simulink model "ProjectArchitecture"  (R2026a)
settings: Solver=VariableStepAuto  StopTime=100
undefined symbols (not defined in the file): Boomgate_Up, Close_Cmd, Dwn, Open, Pedestrian_Lights_On, Traffic_Lights_On
(part 1 of 2)
settings Model: DataDictionary=Architecture_DD.sldd  Creator=jaime  LastModifiedBy=jaime

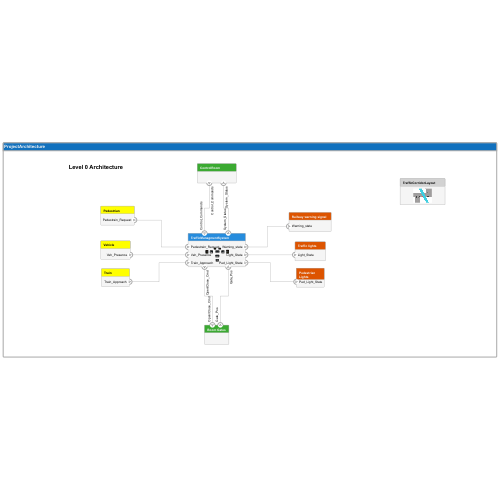
[thumbnail: Simulink's stored preview of the top-level diagram]
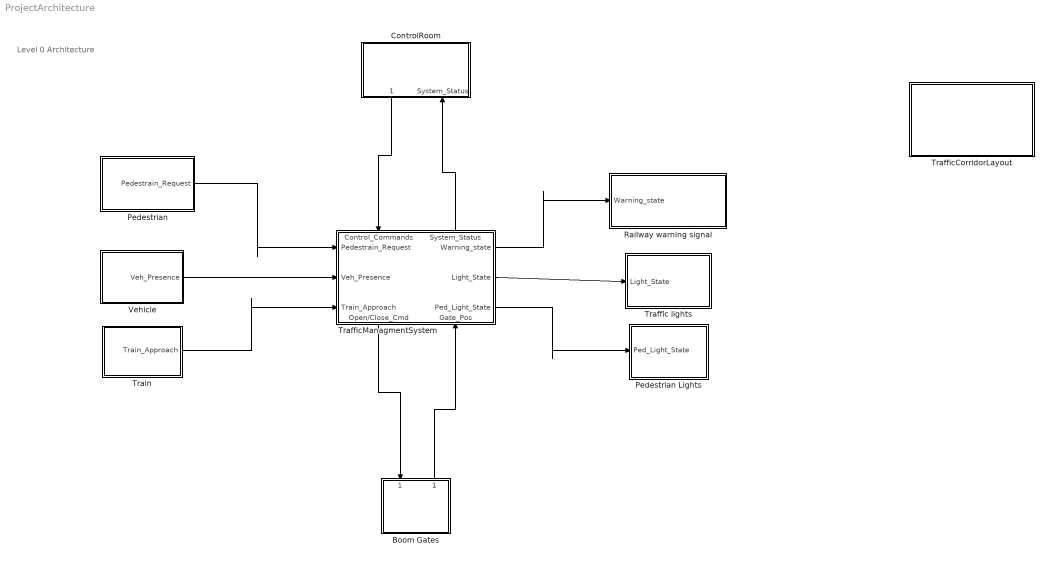
== system ProjectArchitecture ==
  note: Level 0 Architecture
  Boom Gates : Subsystem
      settings: PortSchema="{\"entries\":[{\"content\":{\"headerSize\":26,\"margin\":15,\"minimumSpacing\":25,\"sides\":[{\"content\":{},\"type\":\"ConnectorPlacement.EquallySpacedRectSide\",\"uuid\":\"97ee8f68-7c90-442c-8c58-6fb9a02436b1\"},{\"content\":{\"side\":\"RIGHT\"},\"type\":\"ConnectorPlacement.EquallySpacedRectSide\",\"uuid\":\"273d2447-c6df-49b3-a65a-924db0dbcca5\"},{\"content\":{\"connectorIds\":[\"In1\",\"Out1\"],\"side\":\"TOP\"},\"type\":\"ConnectorPlacement.EquallySpacedRectSide\",\"uuid\":\"83dd206d-8fe2-4459-a401-ead6bb37f785\"}]},\"type\":\"ConnectorPlacement.EquallySpacedConnector\",\"uuid\":\"02b69e8e-5274-42ce-be18-831f28eb2f2d\"}],\"packageUris\":[\"http://schema.mathworks.com/mf0/Connector/R2020b\"],\"version\":\"1.0\"}"
  ControlRoom : Subsystem
      settings: PortSchema="{\"entries\":[{\"content\":{\"headerSize\":26,\"margin\":15,\"minimumSpacing\":25,\"sides\":[{\"content\":{},\"type\":\"ConnectorPlacement.EquallySpacedRectSide\",\"uuid\":\"97ee8f68-7c90-442c-8c58-6fb9a02436b1\"},{\"content\":{\"side\":\"RIGHT\"},\"type\":\"ConnectorPlacement.EquallySpacedRectSide\",\"uuid\":\"273d2447-c6df-49b3-a65a-924db0dbcca5\"},{\"content\":{\"side\":\"TOP\"},\"type\":\"ConnectorPlacement.EquallySpacedRectSide\",\"uuid\":\"83dd206d-8fe2-4459-a401-ead6bb37f785\"},{\"content\":{\"connectorIds\":[\"Out1\",\"In1\"],\"side\":\"BOTTOM\"},\"type\":\"ConnectorPlacement.EquallySpacedRectSide\",\"uuid\":\"7511c607-cb92-42c1-9f90-436e19c4c1f5\"}]},\"type\":\"ConnectorPlacement.EquallySpacedConnector\",\"uuid\":\"02b69e8e-5274-42ce-be18-831f28eb2f2d\"}],\"packageUris\":[\"http://schema.mathworks.com/mf0/Connector/R2020b\"],\"version\":\"1.0\"}"
  Pedestrian : Subsystem
      settings: PortSchema="{\"entries\":[{\"content\":{\"headerSize\":26,\"margin\":15,\"minimumSpacing\":25,\"sides\":[{\"content\":{},\"type\":\"ConnectorPlacement.EquallySpacedRectSide\",\"uuid\":\"97ee8f68-7c90-442c-8c58-6fb9a02436b1\"},{\"content\":{\"connectorIds\":[\"Out1\"],\"side\":\"RIGHT\"},\"type\":\"ConnectorPlacement.EquallySpacedRectSide\",\"uuid\":\"273d2447-c6df-49b3-a65a-924db0dbcca5\"},{\"content\":{\"side\":\"TOP\"},\"type\":\"ConnectorPlacement.EquallySpacedRectSide\",\"uuid\":\"83dd206d-8fe2-4459-a401-ead6bb37f785\"}]},\"type\":\"ConnectorPlacement.EquallySpacedConnector\",\"uuid\":\"02b69e8e-5274-42ce-be18-831f28eb2f2d\"}],\"packageUris\":[\"http://schema.mathworks.com/mf0/Connector/R2020b\"],\"version\":\"1.0\"}"
  Pedestrian Lights : Subsystem
      settings: PortSchema="{\"entries\":[{\"content\":{\"headerSize\":26,\"margin\":15,\"minimumSpacing\":25,\"sides\":[{\"content\":{\"connectorIds\":[\"In1\"]},\"type\":\"ConnectorPlacement.EquallySpacedRectSide\",\"uuid\":\"97ee8f68-7c90-442c-8c58-6fb9a02436b1\"},{\"content\":{\"side\":\"RIGHT\"},\"type\":\"ConnectorPlacement.EquallySpacedRectSide\",\"uuid\":\"273d2447-c6df-49b3-a65a-924db0dbcca5\"},{\"content\":{\"side\":\"TOP\"},\"type\":\"ConnectorPlacement.EquallySpacedRectSide\",\"uuid\":\"83dd206d-8fe2-4459-a401-ead6bb37f785\"}]},\"type\":\"ConnectorPlacement.EquallySpacedConnector\",\"uuid\":\"02b69e8e-5274-42ce-be18-831f28eb2f2d\"}],\"packageUris\":[\"http://schema.mathworks.com/mf0/Connector/R2020b\"],\"version\":\"1.0\"}"
  Railway warning signal : Subsystem
      settings: PortSchema="{\"entries\":[{\"content\":{\"headerSize\":26,\"margin\":15,\"minimumSpacing\":25,\"sides\":[{\"content\":{\"connectorIds\":[\"In1\"]},\"type\":\"ConnectorPlacement.EquallySpacedRectSide\",\"uuid\":\"97ee8f68-7c90-442c-8c58-6fb9a02436b1\"},{\"content\":{\"side\":\"RIGHT\"},\"type\":\"ConnectorPlacement.EquallySpacedRectSide\",\"uuid\":\"273d2447-c6df-49b3-a65a-924db0dbcca5\"},{\"content\":{\"side\":\"TOP\"},\"type\":\"ConnectorPlacement.EquallySpacedRectSide\",\"uuid\":\"83dd206d-8fe2-4459-a401-ead6bb37f785\"}]},\"type\":\"ConnectorPlacement.EquallySpacedConnector\",\"uuid\":\"02b69e8e-5274-42ce-be18-831f28eb2f2d\"}],\"packageUris\":[\"http://schema.mathworks.com/mf0/Connector/R2020b\"],\"version\":\"1.0\"}"
  Traffic lights : Subsystem
      settings: PortSchema="{\"entries\":[{\"content\":{\"headerSize\":26,\"margin\":15,\"minimumSpacing\":25,\"sides\":[{\"content\":{\"connectorIds\":[\"In1\"]},\"type\":\"ConnectorPlacement.EquallySpacedRectSide\",\"uuid\":\"97ee8f68-7c90-442c-8c58-6fb9a02436b1\"},{\"content\":{\"side\":\"RIGHT\"},\"type\":\"ConnectorPlacement.EquallySpacedRectSide\",\"uuid\":\"273d2447-c6df-49b3-a65a-924db0dbcca5\"},{\"content\":{\"side\":\"TOP\"},\"type\":\"ConnectorPlacement.EquallySpacedRectSide\",\"uuid\":\"83dd206d-8fe2-4459-a401-ead6bb37f785\"}]},\"type\":\"ConnectorPlacement.EquallySpacedConnector\",\"uuid\":\"02b69e8e-5274-42ce-be18-831f28eb2f2d\"}],\"packageUris\":[\"http://schema.mathworks.com/mf0/Connector/R2020b\"],\"version\":\"1.0\"}"
  TrafficCorridorLayout : Subsystem
      settings: PortSchema="{\"entries\":[{\"content\":{\"headerSize\":26,\"margin\":15,\"minimumSpacing\":25,\"sides\":[{\"content\":{},\"type\":\"ConnectorPlacement.EquallySpacedRectSide\",\"uuid\":\"5e856c94-202a-4db7-8bb0-19ecc7451e2e\"},{\"content\":{\"side\":\"RIGHT\"},\"type\":\"ConnectorPlacement.EquallySpacedRectSide\",\"uuid\":\"60535048-e66e-4ce0-b527-a8381120427d\"},{\"content\":{\"side\":\"TOP\"},\"type\":\"ConnectorPlacement.EquallySpacedRectSide\",\"uuid\":\"89f0e98b-19cd-4c6c-a057-5a9848434c28\"}]},\"type\":\"ConnectorPlacement.EquallySpacedConnector\",\"uuid\":\"91963807-6f38-48ec-a453-a1c872930595\"}],\"packageUris\":[\"http://schema.mathworks.com/mf0/Connector/R2020b\"],\"version\":\"1.0\"}"
  TrafficManagmentSystem : Subsystem
      settings: PortSchema="{\"entries\":[{\"content\":{\"headerSize\":26,\"margin\":15,\"minimumSpacing\":25,\"sides\":[{\"content\":{\"connectorIds\":[\"In3\",\"In4\",\"In5\"]},\"type\":\"ConnectorPlacement.EquallySpacedRectSide\",\"uuid\":\"97ee8f68-7c90-442c-8c58-6fb9a02436b1\"},{\"content\":{\"connectorIds\":[\"Out1\",\"Out2\",\"Out3\"],\"side\":\"RIGHT\"},\"type\":\"ConnectorPlacement.EquallySpacedRectSide\",\"uuid\":\"273d2447-c6df-49b3-a65a-924db0dbcca5\"},{\"content\":{\"connectorIds\":[\"In2\",\"Out5\"],\"side\":\"TOP\"},\"type\":\"ConnectorPlacement.EquallySpacedRectSide\",\"uuid\":\"83dd206d-8fe2-4459-a401-ead6bb37f785\"},{\"content\":{\"connectorIds\":[\"Out4\",\"In1\"],\"side\":\"BOTTOM\"},\"type\":\"ConnectorPlacement.EquallySpacedRectSide\",\"uuid\":\"d3110f55-67a6-4d73-b0ad-816204b8dc40\"}]},\"type\":\"ConnectorPlacement.EquallySpacedConnector\",\"uuid\":\"02b69e8e-5274-42ce-be18-831f28eb2f2d\"}],\"packageUris\":[\"http://schema.mathworks.com/mf0/Connector/R2020b\"],\"version\":\"1.0\"}"
  Train : Subsystem
      settings: PortSchema="{\"entries\":[{\"content\":{\"headerSize\":26,\"margin\":15,\"minimumSpacing\":25,\"sides\":[{\"content\":{},\"type\":\"ConnectorPlacement.EquallySpacedRectSide\",\"uuid\":\"97ee8f68-7c90-442c-8c58-6fb9a02436b1\"},{\"content\":{\"connectorIds\":[\"Out1\"],\"side\":\"RIGHT\"},\"type\":\"ConnectorPlacement.EquallySpacedRectSide\",\"uuid\":\"273d2447-c6df-49b3-a65a-924db0dbcca5\"},{\"content\":{\"side\":\"TOP\"},\"type\":\"ConnectorPlacement.EquallySpacedRectSide\",\"uuid\":\"83dd206d-8fe2-4459-a401-ead6bb37f785\"}]},\"type\":\"ConnectorPlacement.EquallySpacedConnector\",\"uuid\":\"02b69e8e-5274-42ce-be18-831f28eb2f2d\"}],\"packageUris\":[\"http://schema.mathworks.com/mf0/Connector/R2020b\"],\"version\":\"1.0\"}"
  Vehicle : Subsystem
      settings: PortSchema="{\"entries\":[{\"content\":{\"headerSize\":26,\"margin\":15,\"minimumSpacing\":25,\"sides\":[{\"content\":{},\"type\":\"ConnectorPlacement.EquallySpacedRectSide\",\"uuid\":\"97ee8f68-7c90-442c-8c58-6fb9a02436b1\"},{\"content\":{\"connectorIds\":[\"Out1\"],\"side\":\"RIGHT\"},\"type\":\"ConnectorPlacement.EquallySpacedRectSide\",\"uuid\":\"273d2447-c6df-49b3-a65a-924db0dbcca5\"},{\"content\":{\"side\":\"TOP\"},\"type\":\"ConnectorPlacement.EquallySpacedRectSide\",\"uuid\":\"83dd206d-8fe2-4459-a401-ead6bb37f785\"}]},\"type\":\"ConnectorPlacement.EquallySpacedConnector\",\"uuid\":\"02b69e8e-5274-42ce-be18-831f28eb2f2d\"}],\"packageUris\":[\"http://schema.mathworks.com/mf0/Connector/R2020b\"],\"version\":\"1.0\"}"
  wires:
  Pedestrian/1(Pedestrain_Request) -> TrafficManagmentSystem/3(Pedestrain_Request)
  Train/1(Train_Approach) -> TrafficManagmentSystem/5(Train_Approach)
  ControlRoom/1(Control_Commands) -> TrafficManagmentSystem/2(Control_Commands)
  TrafficManagmentSystem/5(System_Status) -> ControlRoom/1(System_Status)
  TrafficManagmentSystem/4(Open/Close_Cmd) -> Boom Gates/1(Open/Close_Cmd)
  TrafficManagmentSystem/3(Ped_Light_State) -> Pedestrian Lights/1(Ped_Light_State)
  TrafficManagmentSystem/2(Light_State) -> Traffic lights/1(Light_State)
  Boom Gates/1(Gate_Pos) -> TrafficManagmentSystem/1(Gate_Pos)
  TrafficManagmentSystem/1(Warning_state) -> Railway warning signal/1(Warning_state)
  Vehicle/1(Veh_Presence) -> TrafficManagmentSystem/4(Veh_Presence)

== system ProjectArchitecture/Boom Gates ==
  Bus Element In1 : Inport  PortName=Open/Close_Cmd
  Bus Element Out1 : Outport  PortName=Gate_Pos

== system ProjectArchitecture/ControlRoom ==
  Bus Element In1 : Inport  PortName=System_Status
  Bus Element Out1 : Outport  PortName=Control_Commands

== system ProjectArchitecture/Pedestrian ==
  Bus Element Out1 : Outport  PortName=Pedestrain_Request

== system ProjectArchitecture/Pedestrian Lights ==
  Bus Element In1 : Inport  PortName=Ped_Light_State

== system ProjectArchitecture/Railway warning signal ==
  Bus Element In1 : Inport  PortName=Warning_state

== system ProjectArchitecture/Traffic lights ==
  Bus Element In1 : Inport  PortName=Light_State

== system ProjectArchitecture/TrafficCorridorLayout ==

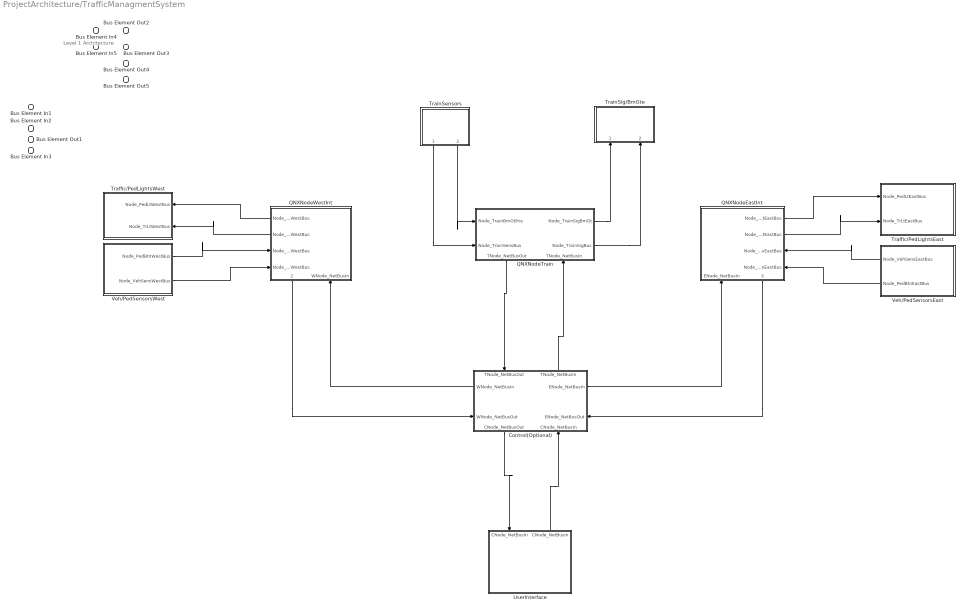
== system ProjectArchitecture/TrafficManagmentSystem ==
  note: Level 1 Architecture
  Bus Element In5 : Inport  PortName=Gate_Pos
  Bus Element In4 : Inport  Port=2  PortName=Control_Commands
  Bus Element In1 : Inport  Port=3  PortName=Pedestrain_Request
  Bus Element In2 : Inport  Port=4  PortName=Veh_Presence
  Bus Element In3 : Inport  Port=5  PortName=Train_Approach
  Control(Optional) : Subsystem
      settings: PortSchema="{\"entries\":[{\"content\":{\"headerSize\":26,\"margin\":15,\"minimumSpacing\":25,\"sides\":[{\"content\":{\"connectorIds\":[\"Out2\",\"In2\"]},\"type\":\"ConnectorPlacement.EquallySpacedRectSide\",\"uuid\":\"5e856c94-202a-4db7-8bb0-19ecc7451e2e\"},{\"content\":{\"connectorIds\":[\"Out3\",\"In3\"],\"side\":\"RIGHT\"},\"type\":\"ConnectorPlacement.EquallySpacedRectSide\",\"uuid\":\"60535048-e66e-4ce0-b527-a8381120427d\"},{\"content\":{\"connectorIds\":[\"In4\",\"Out4\"],\"side\":\"TOP\"},\"type\":\"ConnectorPlacement.EquallySpacedRectSide\",\"uuid\":\"89f0e98b-19cd-4c6c-a057-5a9848434c28\"},{\"content\":{\"connectorIds\":[\"Out1\",\"In1\"],\"side\":\"BOTTOM\"},\"type\":\"ConnectorPlacement.EquallySpacedRectSide\",\"uuid\":\"faeaf1af-5683-4e39-9a46-fc711585bbd4\"}]},\"type\":\"ConnectorPlacement.EquallySpacedConnector\",\"uuid\":\"91963807-6f38-48ec-a453-a1c872930595\"}],\"packageUris\":[\"http://schema.mathworks.com/mf0/Connector/R2020b\"],\"version\":\"1.0\"}"
  QNXNodeEastInt : Subsystem
      settings: PortSchema="{\"entries\":[{\"content\":{\"headerSize\":26,\"margin\":15,\"minimumSpacing\":25,\"sides\":[{\"content\":{},\"type\":\"ConnectorPlacement.EquallySpacedRectSide\",\"uuid\":\"97ee8f68-7c90-442c-8c58-6fb9a02436b1\"},{\"content\":{\"connectorIds\":[\"Out1\",\"Out2\",\"In3\",\"In1\"],\"side\":\"RIGHT\"},\"type\":\"ConnectorPlacement.EquallySpacedRectSide\",\"uuid\":\"273d2447-c6df-49b3-a65a-924db0dbcca5\"},{\"content\":{\"side\":\"TOP\"},\"type\":\"ConnectorPlacement.EquallySpacedRectSide\",\"uuid\":\"83dd206d-8fe2-4459-a401-ead6bb37f785\"},{\"content\":{\"connectorIds\":[\"In2\",\"Out3\"],\"side\":\"BOTTOM\"},\"type\":\"ConnectorPlacement.EquallySpacedRectSide\",\"uuid\":\"1ad8bd89-5dfe-4483-8b48-b0b825829dbd\"}]},\"type\":\"ConnectorPlacement.EquallySpacedConnector\",\"uuid\":\"02b69e8e-5274-42ce-be18-831f28eb2f2d\"}],\"packageUris\":[\"http://schema.mathworks.com/mf0/Connector/R2020b\"],\"version\":\"1.0\"}"
  QNXNodeTrain : Subsystem
      settings: PortSchema="{\"entries\":[{\"content\":{\"headerSize\":26,\"margin\":15,\"minimumSpacing\":25,\"sides\":[{\"content\":{\"connectorIds\":[\"In1\",\"In3\"]},\"type\":\"ConnectorPlacement.EquallySpacedRectSide\",\"uuid\":\"97ee8f68-7c90-442c-8c58-6fb9a02436b1\"},{\"content\":{\"connectorIds\":[\"Out1\",\"Out2\"],\"side\":\"RIGHT\"},\"type\":\"ConnectorPlacement.EquallySpacedRectSide\",\"uuid\":\"273d2447-c6df-49b3-a65a-924db0dbcca5\"},{\"content\":{\"side\":\"TOP\"},\"type\":\"ConnectorPlacement.EquallySpacedRectSide\",\"uuid\":\"83dd206d-8fe2-4459-a401-ead6bb37f785\"},{\"content\":{\"connectorIds\":[\"Out3\",\"In2\"],\"side\":\"BOTTOM\"},\"type\":\"ConnectorPlacement.EquallySpacedRectSide\",\"uuid\":\"71078d88-1727-4f3e-bd9c-f28b6a1550b3\"}]},\"type\":\"ConnectorPlacement.EquallySpacedConnector\",\"uuid\":\"02b69e8e-5274-42ce-be18-831f28eb2f2d\"}],\"packageUris\":[\"http://schema.mathworks.com/mf0/Connector/R2020b\"],\"version\":\"1.0\"}"
  QNXNodeWestInt : Subsystem
      settings: PortSchema="{\"entries\":[{\"content\":{\"headerSize\":26,\"margin\":15,\"minimumSpacing\":25,\"sides\":[{\"content\":{\"connectorIds\":[\"Out1\",\"Out3\",\"In1\",\"In3\"]},\"type\":\"ConnectorPlacement.EquallySpacedRectSide\",\"uuid\":\"97ee8f68-7c90-442c-8c58-6fb9a02436b1\"},{\"content\":{\"side\":\"RIGHT\"},\"type\":\"ConnectorPlacement.EquallySpacedRectSide\",\"uuid\":\"273d2447-c6df-49b3-a65a-924db0dbcca5\"},{\"content\":{\"side\":\"TOP\"},\"type\":\"ConnectorPlacement.EquallySpacedRectSide\",\"uuid\":\"83dd206d-8fe2-4459-a401-ead6bb37f785\"},{\"content\":{\"connectorIds\":[\"Out2\",\"In2\"],\"side\":\"BOTTOM\"},\"type\":\"ConnectorPlacement.EquallySpacedRectSide\",\"uuid\":\"d61255a2-7c77-4b07-b258-3dd7efe5052d\"}]},\"type\":\"ConnectorPlacement.EquallySpacedConnector\",\"uuid\":\"02b69e8e-5274-42ce-be18-831f28eb2f2d\"}],\"packageUris\":[\"http://schema.mathworks.com/mf0/Connector/R2020b\"],\"version\":\"1.0\"}"
  Traffic/PedLightsEast : Subsystem
      settings: PortSchema="{\"entries\":[{\"content\":{\"headerSize\":26,\"margin\":15,\"minimumSpacing\":25,\"sides\":[{\"content\":{\"connectorIds\":[\"In1\",\"In2\"]},\"type\":\"ConnectorPlacement.EquallySpacedRectSide\",\"uuid\":\"97ee8f68-7c90-442c-8c58-6fb9a02436b1\"},{\"content\":{\"side\":\"RIGHT\"},\"type\":\"ConnectorPlacement.EquallySpacedRectSide\",\"uuid\":\"273d2447-c6df-49b3-a65a-924db0dbcca5\"},{\"content\":{\"side\":\"TOP\"},\"type\":\"ConnectorPlacement.EquallySpacedRectSide\",\"uuid\":\"83dd206d-8fe2-4459-a401-ead6bb37f785\"},{\"content\":{\"side\":\"BOTTOM\"},\"type\":\"ConnectorPlacement.EquallySpacedRectSide\",\"uuid\":\"2ab7acb7-b387-4457-9dd3-2605aebb4f9e\"}]},\"type\":\"ConnectorPlacement.EquallySpacedConnector\",\"uuid\":\"02b69e8e-5274-42ce-be18-831f28eb2f2d\"}],\"packageUris\":[\"http://schema.mathworks.com/mf0/Connector/R2020b\"],\"version\":\"1.0\"}"
  Traffic/PedLightsWest : Subsystem
      settings: PortSchema="{\"entries\":[{\"content\":{\"headerSize\":26,\"margin\":15,\"minimumSpacing\":25,\"sides\":[{\"content\":{},\"type\":\"ConnectorPlacement.EquallySpacedRectSide\",\"uuid\":\"97ee8f68-7c90-442c-8c58-6fb9a02436b1\"},{\"content\":{\"connectorIds\":[\"In1\",\"In2\"],\"side\":\"RIGHT\"},\"type\":\"ConnectorPlacement.EquallySpacedRectSide\",\"uuid\":\"273d2447-c6df-49b3-a65a-924db0dbcca5\"},{\"content\":{\"side\":\"TOP\"},\"type\":\"ConnectorPlacement.EquallySpacedRectSide\",\"uuid\":\"83dd206d-8fe2-4459-a401-ead6bb37f785\"},{\"content\":{\"side\":\"BOTTOM\"},\"type\":\"ConnectorPlacement.EquallySpacedRectSide\",\"uuid\":\"b973e172-de59-40eb-a44e-42ad346b123d\"}]},\"type\":\"ConnectorPlacement.EquallySpacedConnector\",\"uuid\":\"02b69e8e-5274-42ce-be18-831f28eb2f2d\"}],\"packageUris\":[\"http://schema.mathworks.com/mf0/Connector/R2020b\"],\"version\":\"1.0\"}"
  TrainSensors : Subsystem
      settings: PortSchema="{\"entries\":[{\"content\":{\"headerSize\":26,\"margin\":15,\"minimumSpacing\":25,\"sides\":[{\"content\":{},\"type\":\"ConnectorPlacement.EquallySpacedRectSide\",\"uuid\":\"97ee8f68-7c90-442c-8c58-6fb9a02436b1\"},{\"content\":{\"side\":\"RIGHT\"},\"type\":\"ConnectorPlacement.EquallySpacedRectSide\",\"uuid\":\"273d2447-c6df-49b3-a65a-924db0dbcca5\"},{\"content\":{\"side\":\"TOP\"},\"type\":\"ConnectorPlacement.EquallySpacedRectSide\",\"uuid\":\"83dd206d-8fe2-4459-a401-ead6bb37f785\"},{\"content\":{\"connectorIds\":[\"Out1\",\"Out2\"],\"side\":\"BOTTOM\"},\"type\":\"ConnectorPlacement.EquallySpacedRectSide\",\"uuid\":\"79500a08-ed4e-4cdc-ae3f-ed43ff6ca98a\"}]},\"type\":\"ConnectorPlacement.EquallySpacedConnector\",\"uuid\":\"02b69e8e-5274-42ce-be18-831f28eb2f2d\"}],\"packageUris\":[\"http://schema.mathworks.com/mf0/Connector/R2020b\"],\"version\":\"1.0\"}"
  TrainSig/BmGte : Subsystem
      settings: PortSchema="{\"entries\":[{\"content\":{\"headerSize\":26,\"margin\":15,\"minimumSpacing\":25,\"sides\":[{\"content\":{},\"type\":\"ConnectorPlacement.EquallySpacedRectSide\",\"uuid\":\"97ee8f68-7c90-442c-8c58-6fb9a02436b1\"},{\"content\":{\"side\":\"RIGHT\"},\"type\":\"ConnectorPlacement.EquallySpacedRectSide\",\"uuid\":\"273d2447-c6df-49b3-a65a-924db0dbcca5\"},{\"content\":{\"side\":\"TOP\"},\"type\":\"ConnectorPlacement.EquallySpacedRectSide\",\"uuid\":\"83dd206d-8fe2-4459-a401-ead6bb37f785\"},{\"content\":{\"connectorIds\":[\"In1\",\"In2\"],\"side\":\"BOTTOM\"},\"type\":\"ConnectorPlacement.EquallySpacedRectSide\",\"uuid\":\"e3797c21-1b15-449b-96ad-f4820117a29f\"}]},\"type\":\"ConnectorPlacement.EquallySpacedConnector\",\"uuid\":\"02b69e8e-5274-42ce-be18-831f28eb2f2d\"}],\"packageUris\":[\"http://schema.mathworks.com/mf0/Connector/R2020b\"],\"version\":\"1.0\"}"
  UserInterface : Subsystem
      settings: PortSchema="{\"entries\":[{\"content\":{\"headerSize\":26,\"margin\":15,\"minimumSpacing\":25,\"sides\":[{\"content\":{},\"type\":\"ConnectorPlacement.EquallySpacedRectSide\",\"uuid\":\"97ee8f68-7c90-442c-8c58-6fb9a02436b1\"},{\"content\":{\"side\":\"RIGHT\"},\"type\":\"ConnectorPlacement.EquallySpacedRectSide\",\"uuid\":\"273d2447-c6df-49b3-a65a-924db0dbcca5\"},{\"content\":{\"connectorIds\":[\"In1\",\"Out1\"],\"side\":\"TOP\"},\"type\":\"ConnectorPlacement.EquallySpacedRectSide\",\"uuid\":\"83dd206d-8fe2-4459-a401-ead6bb37f785\"}]},\"type\":\"ConnectorPlacement.EquallySpacedConnector\",\"uuid\":\"02b69e8e-5274-42ce-be18-831f28eb2f2d\"}],\"packageUris\":[\"http://schema.mathworks.com/mf0/Connector/R2020b\"],\"version\":\"1.0\"}"
  Veh/PedSensorsEast : Subsystem
      settings: PortSchema="{\"entries\":[{\"content\":{\"headerSize\":26,\"margin\":15,\"minimumSpacing\":25,\"sides\":[{\"content\":{\"connectorIds\":[\"Out1\",\"Out2\"]},\"type\":\"ConnectorPlacement.EquallySpacedRectSide\",\"uuid\":\"97ee8f68-7c90-442c-8c58-6fb9a02436b1\"},{\"content\":{\"side\":\"RIGHT\"},\"type\":\"ConnectorPlacement.EquallySpacedRectSide\",\"uuid\":\"273d2447-c6df-49b3-a65a-924db0dbcca5\"},{\"content\":{\"side\":\"TOP\"},\"type\":\"ConnectorPlacement.EquallySpacedRectSide\",\"uuid\":\"83dd206d-8fe2-4459-a401-ead6bb37f785\"}]},\"type\":\"ConnectorPlacement.EquallySpacedConnector\",\"uuid\":\"02b69e8e-5274-42ce-be18-831f28eb2f2d\"}],\"packageUris\":[\"http://schema.mathworks.com/mf0/Connector/R2020b\"],\"version\":\"1.0\"}"
  Veh/PedSensorsWest : Subsystem
      settings: PortSchema="{\"entries\":[{\"content\":{\"headerSize\":26,\"margin\":15,\"minimumSpacing\":25,\"sides\":[{\"content\":{},\"type\":\"ConnectorPlacement.EquallySpacedRectSide\",\"uuid\":\"97ee8f68-7c90-442c-8c58-6fb9a02436b1\"},{\"content\":{\"connectorIds\":[\"Out1\",\"Out2\"],\"side\":\"RIGHT\"},\"type\":\"ConnectorPlacement.EquallySpacedRectSide\",\"uuid\":\"273d2447-c6df-49b3-a65a-924db0dbcca5\"},{\"content\":{\"side\":\"TOP\"},\"type\":\"ConnectorPlacement.EquallySpacedRectSide\",\"uuid\":\"83dd206d-8fe2-4459-a401-ead6bb37f785\"}]},\"type\":\"ConnectorPlacement.EquallySpacedConnector\",\"uuid\":\"02b69e8e-5274-42ce-be18-831f28eb2f2d\"}],\"packageUris\":[\"http://schema.mathworks.com/mf0/Connector/R2020b\"],\"version\":\"1.0\"}"
  Bus Element Out5 : Outport  PortName=Warning_state
  Bus Element Out4 : Outport  Port=2  PortName=Light_State
  Bus Element Out3 : Outport  Port=3  PortName=Ped_Light_State
  Bus Element Out2 : Outport  Port=4  PortName=Open/Close_Cmd
  Bus Element Out1 : Outport  Port=5  PortName=System_Status
  wires:
  TrainSensors/1(Node_TrainSensBus) -> QNXNodeTrain/3(Node_TrainSensBus)
  Veh/PedSensorsWest/2(Node_VehSensWestBus) -> QNXNodeWestInt/3(Node_VehSensWestBus)
  QNXNodeEastInt/2(Node_TrLtEastBus) -> Traffic/PedLightsEast/2(Node_TrLtEastBus)
  Veh/PedSensorsEast/1(Node_VehSensEastBus) -> QNXNodeEastInt/3(Node_VehSensEastBus)
  Veh/PedSensorsEast/2(Node_PedBtnEastBus) -> QNXNodeEastInt/1(Node_PedBtnEastBus)
  Veh/PedSensorsWest/1(Node_PedBtnWestBus) -> QNXNodeWestInt/1(Node_PedBtnWestBus)
  QNXNodeWestInt/3(Node_TrLtWestBus) -> Traffic/PedLightsWest/2(Node_TrLtWestBus)
  QNXNodeTrain/3(TNode_NetBusOut) -> Control(Optional)/4(TNode_NetBusOut)
  Control(Optional)/4(TNode_NetBusIn) -> QNXNodeTrain/2(TNode_NetBusIn)
  Control(Optional)/3(ENode_NetBusIn) -> QNXNodeEastInt/2(ENode_NetBusIn)
  QNXNodeEastInt/3(ENode_NetBusOut) -> Control(Optional)/3(ENode_NetBusOut)
  Control(Optional)/2(WNode_NetBusIn) -> QNXNodeWestInt/2(WNode_NetBusIn)
  QNXNodeWestInt/2(WNode_NetBusOut) -> Control(Optional)/2(WNode_NetBusOut)
  Control(Optional)/1(CNode_NetBusOut) -> UserInterface/1(CNode_NetBusIn)
  UserInterface/1("CNode_NetBusIn ") -> Control(Optional)/1(CNode_NetBusIn)
  QNXNodeWestInt/1(Node_PedLtWestBus) -> Traffic/PedLightsWest/1(Node_PedLtWestBus)
  QNXNodeTrain/2(Node_TrainSigBus) -> TrainSig/BmGte/2(Node_TrainSigBus)
  QNXNodeEastInt/1(Node_PedLtEastBus) -> Traffic/PedLightsEast/1(Node_PedLtEastBus)
  TrainSensors/2(Node_TrainBmGtPos) -> QNXNodeTrain/1(Node_TrainBmGtPos)
  QNXNodeTrain/1(Node_TrainSigBmGt) -> TrainSig/BmGte/1(Node_TrainSigBmGt)

== system ProjectArchitecture/Train ==
  Bus Element Out1 : Outport  PortName=Train_Approach

== system ProjectArchitecture/Vehicle ==
  Bus Element Out1 : Outport  PortName=Veh_Presence

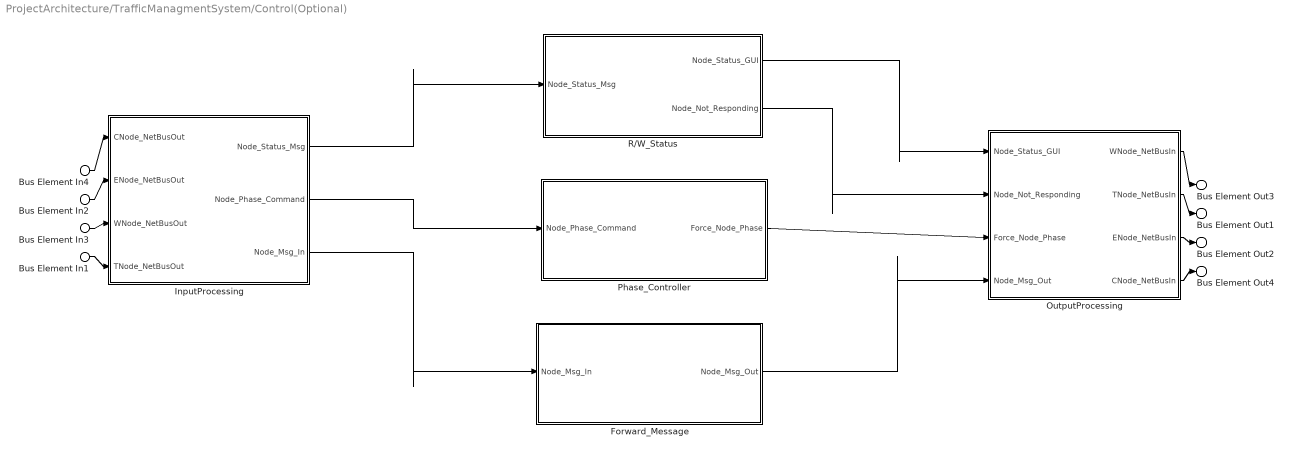
== system ProjectArchitecture/TrafficManagmentSystem/Control(Optional) ==
  Bus Element In4 : Inport  PortName=CNode_NetBusIn
  Bus Element In3 : Inport  Port=2  PortName=WNode_NetBusOut
  Bus Element In2 : Inport  Port=3  PortName=ENode_NetBusOut
  Bus Element In1 : Inport  Port=4  PortName=TNode_NetBusOut
  Forward_Message : Subsystem
      settings: PortSchema="{\"entries\":[{\"content\":{\"headerSize\":26,\"margin\":15,\"minimumSpacing\":25,\"sides\":[{\"content\":{\"connectorIds\":[\"In1\"]},\"type\":\"ConnectorPlacement.EquallySpacedRectSide\",\"uuid\":\"90b308a6-4032-44de-8210-211f4ba540cd\"},{\"content\":{\"connectorIds\":[\"Out1\"],\"side\":\"RIGHT\"},\"type\":\"ConnectorPlacement.EquallySpacedRectSide\",\"uuid\":\"256e3c2d-488f-4744-acae-325334bac20f\"},{\"content\":{\"side\":\"TOP\"},\"type\":\"ConnectorPlacement.EquallySpacedRectSide\",\"uuid\":\"f5068dc7-bb64-4f7e-9eac-58bf28d43dbb\"}]},\"type\":\"ConnectorPlacement.EquallySpacedConnector\",\"uuid\":\"37779c63-bce1-4e78-90a0-aa46b913a6a9\"}],\"packageUris\":[\"http://schema.mathworks.com/mf0/Connector/R2020b\"],\"version\":\"1.0\"}"
  InputProcessing : Subsystem
      settings: PortSchema="{\"entries\":[{\"content\":{\"headerSize\":26,\"margin\":15,\"minimumSpacing\":25,\"sides\":[{\"content\":{\"connectorIds\":[\"In3\",\"In4\",\"In2\",\"In1\"]},\"type\":\"ConnectorPlacement.EquallySpacedRectSide\",\"uuid\":\"3a7ae5c4-38cc-4339-b067-d8e5aa5ceebf\"},{\"content\":{\"connectorIds\":[\"Out1\",\"Out2\",\"Out3\"],\"side\":\"RIGHT\"},\"type\":\"ConnectorPlacement.EquallySpacedRectSide\",\"uuid\":\"7a0e768e-b128-407c-a221-5d8283cba62d\"},{\"content\":{\"side\":\"TOP\"},\"type\":\"ConnectorPlacement.EquallySpacedRectSide\",\"uuid\":\"45545e3e-6bce-40bd-b9a4-cf7cb6bef1ea\"}]},\"type\":\"ConnectorPlacement.EquallySpacedConnector\",\"uuid\":\"469e085b-999a-4159-8aaa-0a4b29cd9c37\"}],\"packageUris\":[\"http://schema.mathworks.com/mf0/Connector/R2020b\"],\"version\":\"1.0\"}"
  OutputProcessing : Subsystem
      settings: PortSchema="{\"entries\":[{\"content\":{\"headerSize\":26,\"margin\":15,\"minimumSpacing\":25,\"sides\":[{\"content\":{\"connectorIds\":[\"In1\",\"In2\",\"In3\",\"In4\"]},\"type\":\"ConnectorPlacement.EquallySpacedRectSide\",\"uuid\":\"90b308a6-4032-44de-8210-211f4ba540cd\"},{\"content\":{\"connectorIds\":[\"Out1\",\"Out2\",\"Out3\",\"Out4\"],\"side\":\"RIGHT\"},\"type\":\"ConnectorPlacement.EquallySpacedRectSide\",\"uuid\":\"256e3c2d-488f-4744-acae-325334bac20f\"},{\"content\":{\"side\":\"TOP\"},\"type\":\"ConnectorPlacement.EquallySpacedRectSide\",\"uuid\":\"f5068dc7-bb64-4f7e-9eac-58bf28d43dbb\"}]},\"type\":\"ConnectorPlacement.EquallySpacedConnector\",\"uuid\":\"37779c63-bce1-4e78-90a0-aa46b913a6a9\"}],\"packageUris\":[\"http://schema.mathworks.com/mf0/Connector/R2020b\"],\"version\":\"1.0\"}"
  Phase_Controller : Subsystem
      settings: PortSchema="{\"entries\":[{\"content\":{\"headerSize\":26,\"margin\":15,\"minimumSpacing\":25,\"sides\":[{\"content\":{\"connectorIds\":[\"In1\"]},\"type\":\"ConnectorPlacement.EquallySpacedRectSide\",\"uuid\":\"90b308a6-4032-44de-8210-211f4ba540cd\"},{\"content\":{\"connectorIds\":[\"Out1\"],\"side\":\"RIGHT\"},\"type\":\"ConnectorPlacement.EquallySpacedRectSide\",\"uuid\":\"256e3c2d-488f-4744-acae-325334bac20f\"},{\"content\":{\"side\":\"TOP\"},\"type\":\"ConnectorPlacement.EquallySpacedRectSide\",\"uuid\":\"f5068dc7-bb64-4f7e-9eac-58bf28d43dbb\"}]},\"type\":\"ConnectorPlacement.EquallySpacedConnector\",\"uuid\":\"37779c63-bce1-4e78-90a0-aa46b913a6a9\"}],\"packageUris\":[\"http://schema.mathworks.com/mf0/Connector/R2020b\"],\"version\":\"1.0\"}"
  R/W_Status : Subsystem
      settings: PortSchema="{\"entries\":[{\"content\":{\"headerSize\":26,\"margin\":15,\"minimumSpacing\":25,\"sides\":[{\"content\":{\"connectorIds\":[\"In1\"]},\"type\":\"ConnectorPlacement.EquallySpacedRectSide\",\"uuid\":\"90b308a6-4032-44de-8210-211f4ba540cd\"},{\"content\":{\"connectorIds\":[\"Out1\",\"Out2\"],\"side\":\"RIGHT\"},\"type\":\"ConnectorPlacement.EquallySpacedRectSide\",\"uuid\":\"256e3c2d-488f-4744-acae-325334bac20f\"},{\"content\":{\"side\":\"TOP\"},\"type\":\"ConnectorPlacement.EquallySpacedRectSide\",\"uuid\":\"f5068dc7-bb64-4f7e-9eac-58bf28d43dbb\"}]},\"type\":\"ConnectorPlacement.EquallySpacedConnector\",\"uuid\":\"37779c63-bce1-4e78-90a0-aa46b913a6a9\"}],\"packageUris\":[\"http://schema.mathworks.com/mf0/Connector/R2020b\"],\"version\":\"1.0\"}"
  Bus Element Out4 : Outport  PortName=CNode_NetBusOut
  Bus Element Out3 : Outport  Port=2  PortName=WNode_NetBusIn
  Bus Element Out2 : Outport  Port=3  PortName=ENode_NetBusIn
  Bus Element Out1 : Outport  Port=4  PortName=TNode_NetBusIn
  wires:
  Bus Element In1/1 -> InputProcessing/1(TNode_NetBusOut)
  Bus Element In3/1 -> InputProcessing/2(WNode_NetBusOut)
  Bus Element In4/1 -> InputProcessing/3(CNode_NetBusOut)
  Bus Element In2/1 -> InputProcessing/4(ENode_NetBusOut)
  OutputProcessing/2(TNode_NetBusIn) -> Bus Element Out1/1
  OutputProcessing/1(WNode_NetBusIn) -> Bus Element Out3/1
  OutputProcessing/3(ENode_NetBusIn) -> Bus Element Out2/1
  OutputProcessing/4(CNode_NetBusIn) -> Bus Element Out4/1
  InputProcessing/1(Node_Status_Msg) -> R/W_Status/1(Node_Status_Msg)
  R/W_Status/1(Node_Status_GUI) -> OutputProcessing/1(Node_Status_GUI)
  R/W_Status/2(Node_Not_Responding) -> OutputProcessing/2(Node_Not_Responding)
  InputProcessing/2(Node_Phase_Command) -> Phase_Controller/1(Node_Phase_Command)
  Phase_Controller/1(Force_Node_Phase) -> OutputProcessing/3(Force_Node_Phase)
  InputProcessing/3(Node_Msg_In) -> Forward_Message/1(Node_Msg_In)
  Forward_Message/1(Node_Msg_Out) -> OutputProcessing/4(Node_Msg_Out)

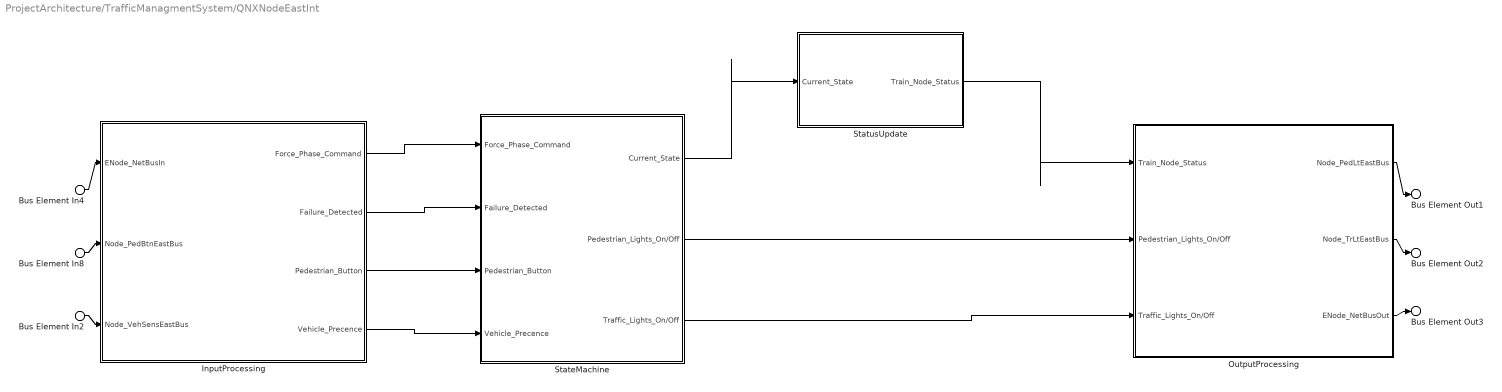
== system ProjectArchitecture/TrafficManagmentSystem/QNXNodeEastInt ==
  Bus Element In8 : Inport  PortName=Node_PedBtnEastBus
  Bus Element In4 : Inport  Port=2  PortName=ENode_NetBusIn
  Bus Element In2 : Inport  Port=3  PortName=Node_VehSensEastBus
  InputProcessing : Subsystem
      settings: PortSchema="{\"entries\":[{\"content\":{\"headerSize\":26,\"margin\":15,\"minimumSpacing\":25,\"sides\":[{\"content\":{\"connectorIds\":[\"In1\",\"In2\",\"In3\"]},\"type\":\"ConnectorPlacement.EquallySpacedRectSide\",\"uuid\":\"3a7ae5c4-38cc-4339-b067-d8e5aa5ceebf\"},{\"content\":{\"connectorIds\":[\"Out1\",\"Out2\",\"Out3\",\"Out4\"],\"side\":\"RIGHT\"},\"type\":\"ConnectorPlacement.EquallySpacedRectSide\",\"uuid\":\"7a0e768e-b128-407c-a221-5d8283cba62d\"},{\"content\":{\"side\":\"TOP\"},\"type\":\"ConnectorPlacement.EquallySpacedRectSide\",\"uuid\":\"45545e3e-6bce-40bd-b9a4-cf7cb6bef1ea\"}]},\"type\":\"ConnectorPlacement.EquallySpacedConnector\",\"uuid\":\"469e085b-999a-4159-8aaa-0a4b29cd9c37\"}],\"packageUris\":[\"http://schema.mathworks.com/mf0/Connector/R2020b\"],\"version\":\"1.0\"}"
  OutputProcessing : Subsystem
      settings: PortSchema="{\"entries\":[{\"content\":{\"headerSize\":26,\"margin\":15,\"minimumSpacing\":25,\"sides\":[{\"content\":{\"connectorIds\":[\"In1\",\"In2\",\"In3\"]},\"type\":\"ConnectorPlacement.EquallySpacedRectSide\",\"uuid\":\"3a7ae5c4-38cc-4339-b067-d8e5aa5ceebf\"},{\"content\":{\"connectorIds\":[\"Out1\",\"Out2\",\"Out3\"],\"side\":\"RIGHT\"},\"type\":\"ConnectorPlacement.EquallySpacedRectSide\",\"uuid\":\"7a0e768e-b128-407c-a221-5d8283cba62d\"},{\"content\":{\"side\":\"TOP\"},\"type\":\"ConnectorPlacement.EquallySpacedRectSide\",\"uuid\":\"45545e3e-6bce-40bd-b9a4-cf7cb6bef1ea\"}]},\"type\":\"ConnectorPlacement.EquallySpacedConnector\",\"uuid\":\"469e085b-999a-4159-8aaa-0a4b29cd9c37\"}],\"packageUris\":[\"http://schema.mathworks.com/mf0/Connector/R2020b\"],\"version\":\"1.0\"}"
  StateMachine : Subsystem
      settings: PortSchema="{\"entries\":[{\"content\":{\"headerSize\":26,\"margin\":15,\"minimumSpacing\":25,\"sides\":[{\"content\":{\"connectorIds\":[\"In1\",\"In2\",\"In3\",\"In4\"]},\"type\":\"ConnectorPlacement.EquallySpacedRectSide\",\"uuid\":\"90b308a6-4032-44de-8210-211f4ba540cd\"},{\"content\":{\"connectorIds\":[\"Out1\",\"Out2\",\"Out3\"],\"side\":\"RIGHT\"},\"type\":\"ConnectorPlacement.EquallySpacedRectSide\",\"uuid\":\"256e3c2d-488f-4744-acae-325334bac20f\"},{\"content\":{\"side\":\"TOP\"},\"type\":\"ConnectorPlacement.EquallySpacedRectSide\",\"uuid\":\"f5068dc7-bb64-4f7e-9eac-58bf28d43dbb\"}]},\"type\":\"ConnectorPlacement.EquallySpacedConnector\",\"uuid\":\"37779c63-bce1-4e78-90a0-aa46b913a6a9\"}],\"packageUris\":[\"http://schema.mathworks.com/mf0/Connector/R2020b\"],\"version\":\"1.0\"}"
  StatusUpdate : Subsystem
      settings: PortSchema="{\"entries\":[{\"content\":{\"headerSize\":26,\"margin\":15,\"minimumSpacing\":25,\"sides\":[{\"content\":{\"connectorIds\":[\"In1\"]},\"type\":\"ConnectorPlacement.EquallySpacedRectSide\",\"uuid\":\"3a7ae5c4-38cc-4339-b067-d8e5aa5ceebf\"},{\"content\":{\"connectorIds\":[\"Out1\"],\"side\":\"RIGHT\"},\"type\":\"ConnectorPlacement.EquallySpacedRectSide\",\"uuid\":\"7a0e768e-b128-407c-a221-5d8283cba62d\"},{\"content\":{\"side\":\"TOP\"},\"type\":\"ConnectorPlacement.EquallySpacedRectSide\",\"uuid\":\"45545e3e-6bce-40bd-b9a4-cf7cb6bef1ea\"}]},\"type\":\"ConnectorPlacement.EquallySpacedConnector\",\"uuid\":\"469e085b-999a-4159-8aaa-0a4b29cd9c37\"}],\"packageUris\":[\"http://schema.mathworks.com/mf0/Connector/R2020b\"],\"version\":\"1.0\"}"
  Bus Element Out1 : Outport  PortName=Node_PedLtEastBus
  Bus Element Out2 : Outport  Port=2  PortName=Node_TrLtEastBus
  Bus Element Out3 : Outport  Port=3  PortName=ENode_NetBusOut
  wires:
  InputProcessing/2(Failure_Detected) -> StateMachine/2(Failure_Detected)
  StateMachine/2(Pedestrian_Lights_On/Off) -> OutputProcessing/2(Pedestrian_Lights_On/Off)
  StatusUpdate/1(Train_Node_Status) -> OutputProcessing/1(Train_Node_Status)
  InputProcessing/1(Force_Phase_Command) -> StateMachine/1(Force_Phase_Command)
  InputProcessing/4(Vehicle_Precence) -> StateMachine/4(Vehicle_Precence)
  StateMachine/1(Current_State) -> StatusUpdate/1(Current_State)
  StateMachine/3(Traffic_Lights_On/Off) -> OutputProcessing/3(Traffic_Lights_On/Off)
  InputProcessing/3(Pedestrian_Button) -> StateMachine/3(Pedestrian_Button)
  OutputProcessing/1(Node_PedLtEastBus) -> Bus Element Out1/1
  OutputProcessing/2(Node_TrLtEastBus) -> Bus Element Out2/1
  OutputProcessing/3(ENode_NetBusOut) -> Bus Element Out3/1
  Bus Element In4/1 -> InputProcessing/1(ENode_NetBusIn)
  Bus Element In8/1 -> InputProcessing/2(Node_PedBtnEastBus)
  Bus Element In2/1 -> InputProcessing/3(Node_VehSensEastBus)

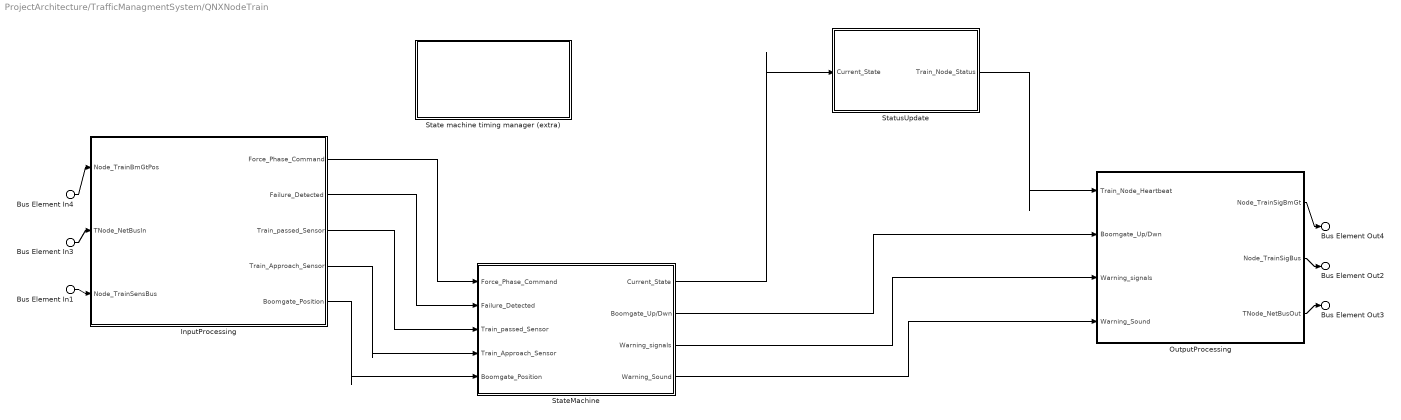
== system ProjectArchitecture/TrafficManagmentSystem/QNXNodeTrain ==
  Bus Element In4 : Inport  PortName=Node_TrainBmGtPos
  Bus Element In3 : Inport  Port=2  PortName=TNode_NetBusIn
  Bus Element In1 : Inport  Port=3  PortName=Node_TrainSensBus
  InputProcessing : Subsystem
      settings: PortSchema="{\"entries\":[{\"content\":{\"headerSize\":26,\"margin\":15,\"minimumSpacing\":25,\"sides\":[{\"content\":{\"connectorIds\":[\"In1\",\"In3\",\"In2\"]},\"type\":\"ConnectorPlacement.EquallySpacedRectSide\",\"uuid\":\"3a7ae5c4-38cc-4339-b067-d8e5aa5ceebf\"},{\"content\":{\"connectorIds\":[\"Out1\",\"Out2\",\"Out3\",\"Out4\",\"Out5\"],\"side\":\"RIGHT\"},\"type\":\"ConnectorPlacement.EquallySpacedRectSide\",\"uuid\":\"7a0e768e-b128-407c-a221-5d8283cba62d\"},{\"content\":{\"side\":\"TOP\"},\"type\":\"ConnectorPlacement.EquallySpacedRectSide\",\"uuid\":\"45545e3e-6bce-40bd-b9a4-cf7cb6bef1ea\"}]},\"type\":\"ConnectorPlacement.EquallySpacedConnector\",\"uuid\":\"469e085b-999a-4159-8aaa-0a4b29cd9c37\"}],\"packageUris\":[\"http://schema.mathworks.com/mf0/Connector/R2020b\"],\"version\":\"1.0\"}"
  OutputProcessing : Subsystem
      settings: PortSchema="{\"entries\":[{\"content\":{\"headerSize\":26,\"margin\":15,\"minimumSpacing\":25,\"sides\":[{\"content\":{\"connectorIds\":[\"In1\",\"In2\",\"In3\",\"In4\"]},\"type\":\"ConnectorPlacement.EquallySpacedRectSide\",\"uuid\":\"3a7ae5c4-38cc-4339-b067-d8e5aa5ceebf\"},{\"content\":{\"connectorIds\":[\"Out1\",\"Out2\",\"Out3\"],\"side\":\"RIGHT\"},\"type\":\"ConnectorPlacement.EquallySpacedRectSide\",\"uuid\":\"7a0e768e-b128-407c-a221-5d8283cba62d\"},{\"content\":{\"side\":\"TOP\"},\"type\":\"ConnectorPlacement.EquallySpacedRectSide\",\"uuid\":\"45545e3e-6bce-40bd-b9a4-cf7cb6bef1ea\"}]},\"type\":\"ConnectorPlacement.EquallySpacedConnector\",\"uuid\":\"469e085b-999a-4159-8aaa-0a4b29cd9c37\"}],\"packageUris\":[\"http://schema.mathworks.com/mf0/Connector/R2020b\"],\"version\":\"1.0\"}"
  State machine timing manager (extra) : Subsystem
      settings: PortSchema="{\"entries\":[{\"content\":{\"headerSize\":26,\"margin\":15,\"minimumSpacing\":25,\"sides\":[{\"content\":{},\"type\":\"ConnectorPlacement.EquallySpacedRectSide\",\"uuid\":\"90b308a6-4032-44de-8210-211f4ba540cd\"},{\"content\":{\"side\":\"RIGHT\"},\"type\":\"ConnectorPlacement.EquallySpacedRectSide\",\"uuid\":\"256e3c2d-488f-4744-acae-325334bac20f\"},{\"content\":{\"side\":\"TOP\"},\"type\":\"ConnectorPlacement.EquallySpacedRectSide\",\"uuid\":\"f5068dc7-bb64-4f7e-9eac-58bf28d43dbb\"}]},\"type\":\"ConnectorPlacement.EquallySpacedConnector\",\"uuid\":\"37779c63-bce1-4e78-90a0-aa46b913a6a9\"}],\"packageUris\":[\"http://schema.mathworks.com/mf0/Connector/R2020b\"],\"version\":\"1.0\"}"
  StateMachine : Subsystem
      settings: PortSchema="{\"entries\":[{\"content\":{\"headerSize\":26,\"margin\":15,\"minimumSpacing\":25,\"sides\":[{\"content\":{\"connectorIds\":[\"In1\",\"In2\",\"In3\",\"In4\",\"In5\"]},\"type\":\"ConnectorPlacement.EquallySpacedRectSide\",\"uuid\":\"90b308a6-4032-44de-8210-211f4ba540cd\"},{\"content\":{\"connectorIds\":[\"Out1\",\"Out2\",\"Out3\",\"Out4\"],\"side\":\"RIGHT\"},\"type\":\"ConnectorPlacement.EquallySpacedRectSide\",\"uuid\":\"256e3c2d-488f-4744-acae-325334bac20f\"},{\"content\":{\"side\":\"TOP\"},\"type\":\"ConnectorPlacement.EquallySpacedRectSide\",\"uuid\":\"f5068dc7-bb64-4f7e-9eac-58bf28d43dbb\"}]},\"type\":\"ConnectorPlacement.EquallySpacedConnector\",\"uuid\":\"37779c63-bce1-4e78-90a0-aa46b913a6a9\"}],\"packageUris\":[\"http://schema.mathworks.com/mf0/Connector/R2020b\"],\"version\":\"1.0\"}"
  StatusUpdate : Subsystem
      settings: PortSchema="{\"entries\":[{\"content\":{\"headerSize\":26,\"margin\":15,\"minimumSpacing\":25,\"sides\":[{\"content\":{\"connectorIds\":[\"In1\"]},\"type\":\"ConnectorPlacement.EquallySpacedRectSide\",\"uuid\":\"3a7ae5c4-38cc-4339-b067-d8e5aa5ceebf\"},{\"content\":{\"connectorIds\":[\"Out1\"],\"side\":\"RIGHT\"},\"type\":\"ConnectorPlacement.EquallySpacedRectSide\",\"uuid\":\"7a0e768e-b128-407c-a221-5d8283cba62d\"},{\"content\":{\"side\":\"TOP\"},\"type\":\"ConnectorPlacement.EquallySpacedRectSide\",\"uuid\":\"45545e3e-6bce-40bd-b9a4-cf7cb6bef1ea\"}]},\"type\":\"ConnectorPlacement.EquallySpacedConnector\",\"uuid\":\"469e085b-999a-4159-8aaa-0a4b29cd9c37\"}],\"packageUris\":[\"http://schema.mathworks.com/mf0/Connector/R2020b\"],\"version\":\"1.0\"}"
  Bus Element Out4 : Outport  PortName=Node_TrainSigBmGt
  Bus Element Out2 : Outport  Port=2  PortName=Node_TrainSigBus
  Bus Element Out3 : Outport  Port=3  PortName=TNode_NetBusOut
  wires:
  Bus Element In1/1 -> InputProcessing/2(Node_TrainSensBus)
  Bus Element In3/1 -> InputProcessing/3(TNode_NetBusIn)
  OutputProcessing/2(Node_TrainSigBus) -> Bus Element Out2/1
  OutputProcessing/3(TNode_NetBusOut) -> Bus Element Out3/1
  StatusUpdate/1(Train_Node_Status) -> OutputProcessing/1(Train_Node_Heartbeat)
  Bus Element In4/1 -> InputProcessing/1(Node_TrainBmGtPos)
  OutputProcessing/1(Node_TrainSigBmGt) -> Bus Element Out4/1
  InputProcessing/3(Train_passed_Sensor) -> StateMachine/3(Train_passed_Sensor)
  InputProcessing/4(Train_Approach_Sensor) -> StateMachine/4(Train_Approach_Sensor)
  InputProcessing/5(Boomgate_Position) -> StateMachine/5(Boomgate_Position)
  InputProcessing/2(Failure_Detected) -> StateMachine/2(Failure_Detected)
  InputProcessing/1(Force_Phase_Command) -> StateMachine/1(Force_Phase_Command)
  StateMachine/1(Current_State) -> StatusUpdate/1(Current_State)
  StateMachine/2(Boomgate_Up/Dwn) -> OutputProcessing/2(Boomgate_Up/Dwn)
  StateMachine/3(Warning_signals) -> OutputProcessing/3(Warning_signals)
  StateMachine/4(Warning_Sound) -> OutputProcessing/4(Warning_Sound)

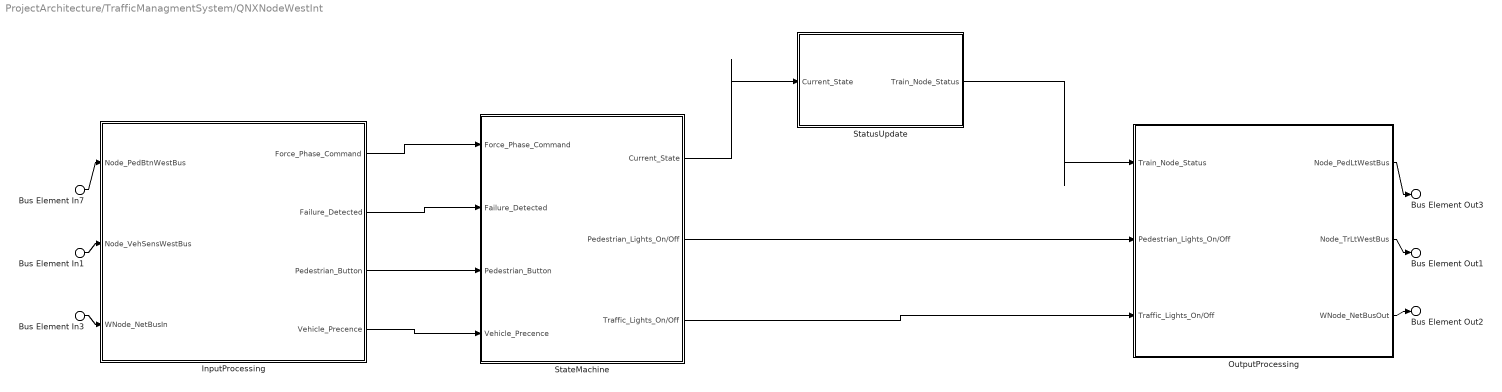
== system ProjectArchitecture/TrafficManagmentSystem/QNXNodeWestInt ==
  Bus Element In7 : Inport  PortName=Node_PedBtnWestBus
  Bus Element In3 : Inport  Port=2  PortName=WNode_NetBusIn
  Bus Element In1 : Inport  Port=3  PortName=Node_VehSensWestBus
  InputProcessing : Subsystem
      settings: PortSchema="{\"entries\":[{\"content\":{\"headerSize\":26,\"margin\":15,\"minimumSpacing\":25,\"sides\":[{\"content\":{\"connectorIds\":[\"In1\",\"In2\",\"In3\"]},\"type\":\"ConnectorPlacement.EquallySpacedRectSide\",\"uuid\":\"3a7ae5c4-38cc-4339-b067-d8e5aa5ceebf\"},{\"content\":{\"connectorIds\":[\"Out1\",\"Out2\",\"Out3\",\"Out4\"],\"side\":\"RIGHT\"},\"type\":\"ConnectorPlacement.EquallySpacedRectSide\",\"uuid\":\"7a0e768e-b128-407c-a221-5d8283cba62d\"},{\"content\":{\"side\":\"TOP\"},\"type\":\"ConnectorPlacement.EquallySpacedRectSide\",\"uuid\":\"45545e3e-6bce-40bd-b9a4-cf7cb6bef1ea\"}]},\"type\":\"ConnectorPlacement.EquallySpacedConnector\",\"uuid\":\"469e085b-999a-4159-8aaa-0a4b29cd9c37\"}],\"packageUris\":[\"http://schema.mathworks.com/mf0/Connector/R2020b\"],\"version\":\"1.0\"}"
  OutputProcessing : Subsystem
      settings: PortSchema="{\"entries\":[{\"content\":{\"headerSize\":26,\"margin\":15,\"minimumSpacing\":25,\"sides\":[{\"content\":{\"connectorIds\":[\"In1\",\"In2\",\"In3\"]},\"type\":\"ConnectorPlacement.EquallySpacedRectSide\",\"uuid\":\"3a7ae5c4-38cc-4339-b067-d8e5aa5ceebf\"},{\"content\":{\"connectorIds\":[\"Out1\",\"Out2\",\"Out3\"],\"side\":\"RIGHT\"},\"type\":\"ConnectorPlacement.EquallySpacedRectSide\",\"uuid\":\"7a0e768e-b128-407c-a221-5d8283cba62d\"},{\"content\":{\"side\":\"TOP\"},\"type\":\"ConnectorPlacement.EquallySpacedRectSide\",\"uuid\":\"45545e3e-6bce-40bd-b9a4-cf7cb6bef1ea\"}]},\"type\":\"ConnectorPlacement.EquallySpacedConnector\",\"uuid\":\"469e085b-999a-4159-8aaa-0a4b29cd9c37\"}],\"packageUris\":[\"http://schema.mathworks.com/mf0/Connector/R2020b\"],\"version\":\"1.0\"}"
  StateMachine : Subsystem
      settings: PortSchema="{\"entries\":[{\"content\":{\"headerSize\":26,\"margin\":15,\"minimumSpacing\":25,\"sides\":[{\"content\":{\"connectorIds\":[\"In1\",\"In2\",\"In3\",\"In4\"]},\"type\":\"ConnectorPlacement.EquallySpacedRectSide\",\"uuid\":\"90b308a6-4032-44de-8210-211f4ba540cd\"},{\"content\":{\"connectorIds\":[\"Out1\",\"Out2\",\"Out3\"],\"side\":\"RIGHT\"},\"type\":\"ConnectorPlacement.EquallySpacedRectSide\",\"uuid\":\"256e3c2d-488f-4744-acae-325334bac20f\"},{\"content\":{\"side\":\"TOP\"},\"type\":\"ConnectorPlacement.EquallySpacedRectSide\",\"uuid\":\"f5068dc7-bb64-4f7e-9eac-58bf28d43dbb\"}]},\"type\":\"ConnectorPlacement.EquallySpacedConnector\",\"uuid\":\"37779c63-bce1-4e78-90a0-aa46b913a6a9\"}],\"packageUris\":[\"http://schema.mathworks.com/mf0/Connector/R2020b\"],\"version\":\"1.0\"}"
  StatusUpdate : Subsystem
      settings: PortSchema="{\"entries\":[{\"content\":{\"headerSize\":26,\"margin\":15,\"minimumSpacing\":25,\"sides\":[{\"content\":{\"connectorIds\":[\"In1\"]},\"type\":\"ConnectorPlacement.EquallySpacedRectSide\",\"uuid\":\"3a7ae5c4-38cc-4339-b067-d8e5aa5ceebf\"},{\"content\":{\"connectorIds\":[\"Out1\"],\"side\":\"RIGHT\"},\"type\":\"ConnectorPlacement.EquallySpacedRectSide\",\"uuid\":\"7a0e768e-b128-407c-a221-5d8283cba62d\"},{\"content\":{\"side\":\"TOP\"},\"type\":\"ConnectorPlacement.EquallySpacedRectSide\",\"uuid\":\"45545e3e-6bce-40bd-b9a4-cf7cb6bef1ea\"}]},\"type\":\"ConnectorPlacement.EquallySpacedConnector\",\"uuid\":\"469e085b-999a-4159-8aaa-0a4b29cd9c37\"}],\"packageUris\":[\"http://schema.mathworks.com/mf0/Connector/R2020b\"],\"version\":\"1.0\"}"
  Bus Element Out3 : Outport  PortName=Node_PedLtWestBus
  Bus Element Out2 : Outport  Port=2  PortName=WNode_NetBusOut
  Bus Element Out1 : Outport  Port=3  PortName=Node_TrLtWestBus
  wires:
  Bus Element In7/1 -> InputProcessing/1(Node_PedBtnWestBus)
  Bus Element In1/1 -> InputProcessing/2(Node_VehSensWestBus)
  Bus Element In3/1 -> InputProcessing/3(WNode_NetBusIn)
  OutputProcessing/1(Node_PedLtWestBus) -> Bus Element Out3/1
  OutputProcessing/2(Node_TrLtWestBus) -> Bus Element Out1/1
  OutputProcessing/3(WNode_NetBusOut) -> Bus Element Out2/1
  StatusUpdate/1(Train_Node_Status) -> OutputProcessing/1(Train_Node_Status)
  StateMachine/1(Current_State) -> StatusUpdate/1(Current_State)
  InputProcessing/3(Pedestrian_Button) -> StateMachine/3(Pedestrian_Button)
  InputProcessing/4(Vehicle_Precence) -> StateMachine/4(Vehicle_Precence)
  InputProcessing/1(Force_Phase_Command) -> StateMachine/1(Force_Phase_Command)
  InputProcessing/2(Failure_Detected) -> StateMachine/2(Failure_Detected)
  StateMachine/2(Pedestrian_Lights_On/Off) -> OutputProcessing/2(Pedestrian_Lights_On/Off)
  StateMachine/3(Traffic_Lights_On/Off) -> OutputProcessing/3(Traffic_Lights_On/Off)

== system ProjectArchitecture/TrafficManagmentSystem/Traffic//PedLightsEast ==
  Bus Element In2 : Inport  PortName=Node_PedLtEastBus
  Bus Element In1 : Inport  Port=2  PortName=Node_TrLtEastBus

== system ProjectArchitecture/TrafficManagmentSystem/Traffic//PedLightsWest ==
  Bus Element In1 : Inport  PortName=Node_PedLtWestBus
  Bus Element In2 : Inport  Port=2  PortName=Node_TrLtWestBus

== system ProjectArchitecture/TrafficManagmentSystem/TrainSensors ==
  Bus Element Out1 : Outport  PortName=Node_TrainSensBus
  Bus Element Out2 : Outport  Port=2  PortName=Node_TrainBmGtPos

== system ProjectArchitecture/TrafficManagmentSystem/TrainSig//BmGte ==
  Bus Element In2 : Inport  PortName=Node_TrainSigBmGt
  Bus Element In1 : Inport  Port=2  PortName=Node_TrainSigBus

== system ProjectArchitecture/TrafficManagmentSystem/UserInterface ==
  note: Level 2 Architecture
  Bus Element In2 : Inport  PortName=CNode_NetBusIn
  InputProcessing : Subsystem
      settings: PortSchema="{\"entries\":[{\"content\":{\"headerSize\":26,\"margin\":15,\"minimumSpacing\":25,\"sides\":[{\"content\":{\"connectorIds\":[\"In1\"]},\"type\":\"ConnectorPlacement.EquallySpacedRectSide\",\"uuid\":\"3363a15c-2c5a-4259-9d43-344454abad48\"},{\"content\":{\"connectorIds\":[\"Out1\"],\"side\":\"RIGHT\"},\"type\":\"ConnectorPlacement.EquallySpacedRectSide\",\"uuid\":\"6d0ff110-eb27-48d2-a755-ec8de2fec90e\"},{\"content\":{\"side\":\"TOP\"},\"type\":\"ConnectorPlacement.EquallySpacedRectSide\",\"uuid\":\"9712bee6-cfad-4c3b-895d-65406f34516c\"}]},\"type\":\"ConnectorPlacement.EquallySpacedConnector\",\"uuid\":\"644a2397-9f24-420a-8566-3b041c1f64bb\"}],\"packageUris\":[\"http://schema.mathworks.com/mf0/Connector/R2020b\"],\"version\":\"1.0\"}"
  Interface (TBD) : Subsystem
      settings: PortSchema="{\"entries\":[{\"content\":{\"headerSize\":26,\"margin\":15,\"minimumSpacing\":25,\"sides\":[{\"content\":{\"connectorIds\":[\"In1\"]},\"type\":\"ConnectorPlacement.EquallySpacedRectSide\",\"uuid\":\"90b308a6-4032-44de-8210-211f4ba540cd\"},{\"content\":{\"connectorIds\":[\"Out1\",\"Out2\"],\"side\":\"RIGHT\"},\"type\":\"ConnectorPlacement.EquallySpacedRectSide\",\"uuid\":\"256e3c2d-488f-4744-acae-325334bac20f\"},{\"content\":{\"side\":\"TOP\"},\"type\":\"ConnectorPlacement.EquallySpacedRectSide\",\"uuid\":\"f5068dc7-bb64-4f7e-9eac-58bf28d43dbb\"}]},\"type\":\"ConnectorPlacement.EquallySpacedConnector\",\"uuid\":\"37779c63-bce1-4e78-90a0-aa46b913a6a9\"}],\"packageUris\":[\"http://schema.mathworks.com/mf0/Connector/R2020b\"],\"version\":\"1.0\"}"
  OutputProcessing : Subsystem
      settings: PortSchema="{\"entries\":[{\"content\":{\"headerSize\":26,\"margin\":15,\"minimumSpacing\":25,\"sides\":[{\"content\":{\"connectorIds\":[\"In1\",\"In2\"]},\"type\":\"ConnectorPlacement.EquallySpacedRectSide\",\"uuid\":\"3363a15c-2c5a-4259-9d43-344454abad48\"},{\"content\":{\"connectorIds\":[\"Out1\"],\"side\":\"RIGHT\"},\"type\":\"ConnectorPlacement.EquallySpacedRectSide\",\"uuid\":\"6d0ff110-eb27-48d2-a755-ec8de2fec90e\"},{\"content\":{\"side\":\"TOP\"},\"type\":\"ConnectorPlacement.EquallySpacedRectSide\",\"uuid\":\"9712bee6-cfad-4c3b-895d-65406f34516c\"}]},\"type\":\"ConnectorPlacement.EquallySpacedConnector\",\"uuid\":\"644a2397-9f24-420a-8566-3b041c1f64bb\"}],\"packageUris\":[\"http://schema.mathworks.com/mf0/Connector/R2020b\"],\"version\":\"1.0\"}"
  StatusUpdate : Subsystem
      settings: PortSchema="{\"entries\":[{\"content\":{\"headerSize\":26,\"margin\":15,\"minimumSpacing\":25,\"sides\":[{\"content\":{\"connectorIds\":[\"In1\"]},\"type\":\"ConnectorPlacement.EquallySpacedRectSide\",\"uuid\":\"3a7ae5c4-38cc-4339-b067-d8e5aa5ceebf\"},{\"content\":{\"connectorIds\":[\"Out1\"],\"side\":\"RIGHT\"},\"type\":\"ConnectorPlacement.EquallySpacedRectSide\",\"uuid\":\"7a0e768e-b128-407c-a221-5d8283cba62d\"},{\"content\":{\"side\":\"TOP\"},\"type\":\"ConnectorPlacement.EquallySpacedRectSide\",\"uuid\":\"45545e3e-6bce-40bd-b9a4-cf7cb6bef1ea\"}]},\"type\":\"ConnectorPlacement.EquallySpacedConnector\",\"uuid\":\"469e085b-999a-4159-8aaa-0a4b29cd9c37\"}],\"packageUris\":[\"http://schema.mathworks.com/mf0/Connector/R2020b\"],\"version\":\"1.0\"}"
  Bus Element Out2 : Outport  PortName=CNode_NetBusIn
  wires:
  Bus Element In2/1 -> InputProcessing/1(CNode_NetBusIn)
  OutputProcessing/1(CNode_NetBusOut) -> Bus Element Out2/1
  Interface (TBD)/1(Current_State) -> StatusUpdate/1(Current_State)
  StatusUpdate/1(UsrInt_Node_Status) -> OutputProcessing/1(UsrInt_Node_Status)
  InputProcessing/1(Display_Info) -> Interface (TBD)/1(Display_Info)
  Interface (TBD)/2(Command_Out) -> OutputProcessing/2(Command_Out)

== system ProjectArchitecture/TrafficManagmentSystem/Veh//PedSensorsEast ==
  Bus Element Out1 : Outport  PortName=Node_VehSensEastBus
  Bus Element Out2 : Outport  Port=2  PortName=Node_PedBtnEastBus

== system ProjectArchitecture/TrafficManagmentSystem/Veh//PedSensorsWest ==
  Bus Element Out2 : Outport  PortName=Node_PedBtnWestBus
  Bus Element Out1 : Outport  Port=2  PortName=Node_VehSensWestBus

== system ProjectArchitecture/TrafficManagmentSystem/Control(Optional)/Forward_Message ==
  Bus Element In1 : Inport  PortName=Node_Msg_In
  Bus Element Out1 : Outport  PortName=Node_Msg_Out

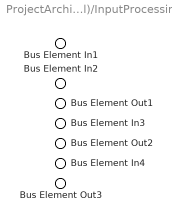
== system ProjectArchitecture/TrafficManagmentSystem/Control(Optional)/InputProcessing ==
  Bus Element In1 : Inport  PortName=TNode_NetBusOut
  Bus Element In2 : Inport  Port=2  PortName=WNode_NetBusOut
  Bus Element In3 : Inport  Port=3  PortName=CNode_NetBusOut
  Bus Element In4 : Inport  Port=4  PortName=ENode_NetBusOut
  Bus Element Out1 : Outport  PortName=Node_Status_Msg
  Bus Element Out2 : Outport  Port=2  PortName=Node_Phase_Command
  Bus Element Out3 : Outport  Port=3  PortName=Node_Msg_In

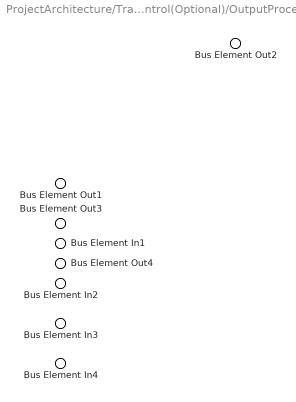
== system ProjectArchitecture/TrafficManagmentSystem/Control(Optional)/OutputProcessing ==
  Bus Element In1 : Inport  PortName=Node_Status_GUI
  Bus Element In2 : Inport  Port=2  PortName=Node_Not_Responding
  Bus Element In3 : Inport  Port=3  PortName=Force_Node_Phase
  Bus Element In4 : Inport  Port=4  PortName=Node_Msg_Out
  Bus Element Out2 : Outport  PortName=WNode_NetBusIn
  Bus Element Out1 : Outport  Port=2  PortName=TNode_NetBusIn
  Bus Element Out3 : Outport  Port=3  PortName=ENode_NetBusIn
  Bus Element Out4 : Outport  Port=4  PortName=CNode_NetBusIn

== system ProjectArchitecture/TrafficManagmentSystem/Control(Optional)/Phase_Controller ==
  Bus Element In1 : Inport  PortName=Node_Phase_Command
  Bus Element Out1 : Outport  PortName=Force_Node_Phase
